simulink model "Model_Mk2"  (R2024a)
settings: Solver=VariableStepAuto  StartTime=startTime  StopTime=stopTime  FixedStep=1e-4  RelTol=1e-9  AbsTol=1e-9  EnableMultiTasking=on
model workspace (MAT data in the model file):
  Kset = [-2.00916512617e-14 -2.1396164685e-13 1645.65145003 1.10700309911e-13 0.064606154931 -1.15620600709 -2.35613942722e-12 1.21905689036 1.1835423475 0.0960813361903 -1.05646659933e-12 0.256355277786 ... (180 elements, 4x15x3)]
  MOI = [0.25  0.023  -0.0888; 0.023  0.5  0.097345; -0.0888  0.097345  0.5]
  betaInputDelay = 0.001
  discretize_interval = 0.0025
  g = 9.81
  gammaInputDelay = 0.001
  inputLimits = [-0.261799387799  0.261799387799; -0.261799387799  0.261799387799; 0  100; -0.1  0.1]
  l = 0.5
  m = 5
  q1 = [0.506236006596; 0.0473671727454; 0.176776695297]
  startTime = 0
  stopTime = 15
  tSegs = [0 7.5 15]
  t_set = [0 0.000750075007501 0.001500150015 0.0022502250225 0.00300030003 0.0037503750375 0.004500450045 0.00525052505251 0.00600060006001 0.00675067506751 0.00750075007501 0.00825082508251 ... (19999 elements, 1x19999)]
  throttleConsts = [71.0072; 0.0504; 67.9056]
  u_set = [-0.261799387799 0.261799387799 0 -0.1 -0.261799387799 0.261799387799 0 -0.1 -0.261799387799 0.261799387799 0 -0.1 ... (79996 elements, 4x19999)]
  x1 = [10; 5; 5; 0; 0; 0; 0.506236006596; 0.0473671727454; 0.176776695297; 0; 0; 0]
  x_set = [10 5 5 0 0 0 0.506236006596 0.0473671727454 0.176776695297 0 0 0 ... (239988 elements, 12x19999)]
undefined symbols (not defined in the file): DiscIntNeverNeededParam
libraries: matrix_library x2, sharedtransform x2, aerolibutil x1, vrlib x1
(part 1 of 2)
settings Model: Creator=davis
settings SolverCC: ZeroCrossAlgorithm=Adaptive  PositivePriorityOrder=on
settings DataIOCC: SaveFormat=Array  SignalLogging=off  DSMLogging=off  ReturnWorkspaceOutputs=off
settings OptimizationCC: DefaultParameterBehavior=Inlined  EnhancedBackFolding=on  PassReuseOutputArgsAs=Individual arguments  ZeroExternalMemoryAtStartup=off  ZeroInternalMemoryAtStartup=off  MaxStackSize=64  OptimizeBlockOrder=speed  DifferentSizesBufferReuse=on  OptimizationCustomize=off  EfficientTunableParamExpr=on
settings DebuggingCC: IgnoredZcDiagnostic=none  ParameterTunabilityLossMsg=error  UnconnectedInputMsg=warning  UnconnectedOutputMsg=warning  UnconnectedLineMsg=warning
settings HardwareCC: ProdBitPerPointer=32  ProdBitPerSizeT=32  ProdBitPerPtrDiffT=32  ProdLargestAtomicInteger=Long  ProdLargestAtomicFloat=Double  ProdWordSize=32  ProdHWDeviceType=ARM Compatible->ARM Cortex-M  HardwareBoardFeatureSet=SoCBlockset
settings ModelReferenceCC: UpdateModelReferenceTargets=Force  EnableRefExpFcnMdlSchedulingChecks=on  ModelReferenceNumInstancesAllowed=Single
settings SFSimCC: MATLABDynamicMemAlloc=off
settings RTWCC: Description=Embedded Coder  SystemTargetFile=ert.tlc  TemplateMakefile=ert_default_tmf  GPUComputeCapability=3.5  DLArmComputeVersion=19.05
settings CodeAppCC: ForceParamTrailComments=on  IgnoreCustomStorageClasses=off  OperatorAnnotations=on  SimulinkDataObjDesc=on  SFDataObjDesc=on  InsertBlockDesc=on
settings ERTTargetCC: ERTCustomFileTemplate=example_file_process.tlc

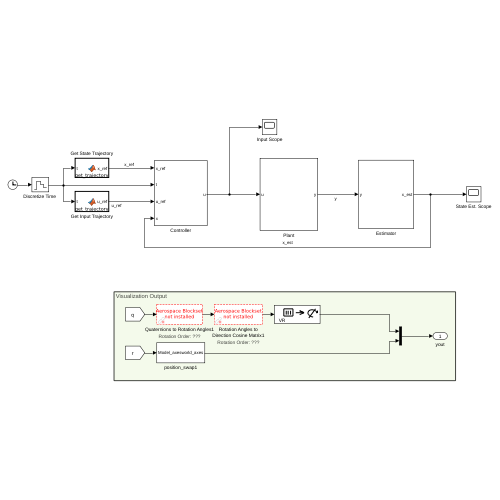
[thumbnail: Simulink's stored preview of the top-level diagram]
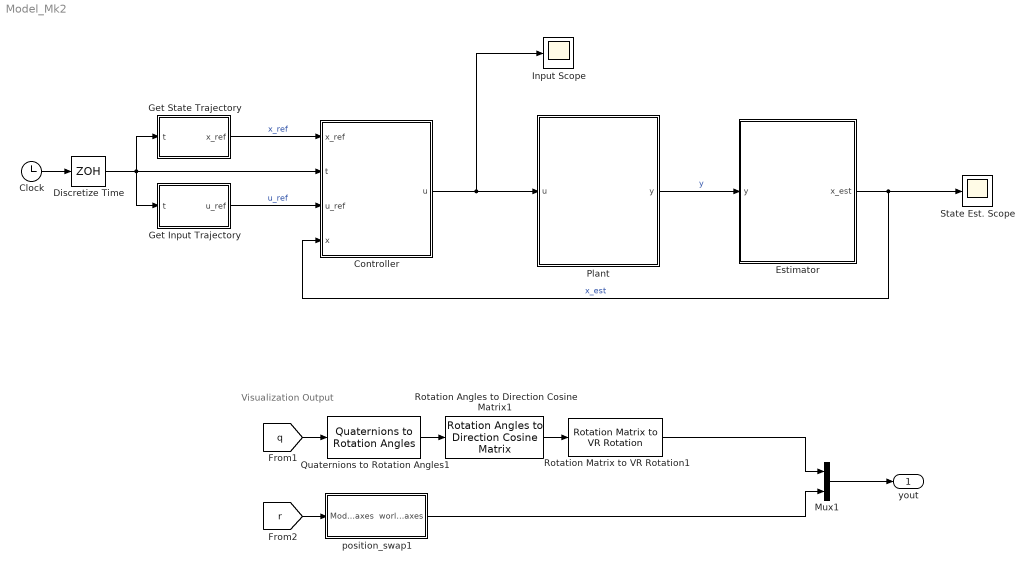
== system Model_Mk2 ==
  note: Visualization Output
  Clock : Clock
  Controller : Subsystem
  "Discretize Time " : ZeroOrderHold  SampleTime=discretize_interval
  Estimator : Subsystem
  Get Input Trajectory : MATLAB Function  TreatAsAtomicUnit=on
  Get State Trajectory : MATLAB Function  TreatAsAtomicUnit=on
  Input Scope : Scope
  Mux1 : Mux  Inputs=2
  Plant : Subsystem
  Quaternions to Rotation Angles1 : sharedtransform/Quaternions to Rotation Angles  rotationOrder=ZYX  aMode=aMode
  Rotation Angles to Direction Cosine Matrix1 : sharedtransform/Rotation Angles to Direction Cosine Matrix  rotationOrder=ZYX  aMode=aMode
  Rotation Matrix to VR Rotation1 : vrlib/Utilities/Rotation Matrix to VR Rotation  maxzero=1e-12
  State Est. Scope : Scope
  position_swap1 : Subsystem
  yout : Outport
  wires:
  Plant/1(y) -> Estimator/1(y)  "y"
  Estimator/1(x_est) -> Controller/4(x), State Est. Scope/1  "x_est"
  Clock/1 -> "Discretize Time "/1
  "Discretize Time "/1 -> Get Input Trajectory/1(t), Controller/2(t), Get State Trajectory/1(t)
  Controller/1(u) -> Input Scope/1, Plant/1(u)
  Get State Trajectory/1(x_ref) -> Controller/1(x_ref)  "x_ref"
  Get Input Trajectory/1(u_ref) -> Controller/3(u_ref)  "u_ref"
  Rotation Angles to Direction Cosine Matrix1/1 -> Rotation Matrix to VR Rotation1/1
  Rotation Matrix to VR Rotation1/1 -> Mux1/1
  Quaternions to Rotation Angles1/1 -> Rotation Angles to Direction Cosine Matrix1/1
  [q] -> Quaternions to Rotation Angles1/1
  [r] -> position_swap1/1(Model_axes)
  Mux1/1 -> yout/1
  position_swap1/1(world_axes) -> Mux1/2
